simulink library "Word_Multiplexers_Lib"  (Simulink 8.7)
settings: Solver=ode45  StartTime=0.0  StopTime=10.0  RelTol=1e-3
(part 1 of 3)
settings Model: Creator=uzivatel  LastModifiedBy=Jozko Mrkvicka

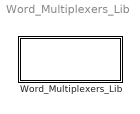
== system Word_Multiplexers_Lib ==
  Word_Multiplexers_Lib : Subsystem

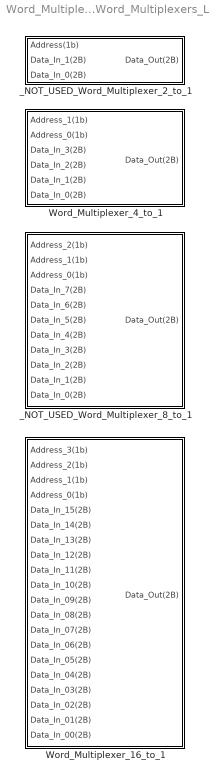
== system Word_Multiplexers_Lib/Word_Multiplexers_Lib ==
  Word_Multiplexer_16_to_1 : Subsystem
  Word_Multiplexer_4_to_1 : Subsystem
  _NOT_USED_Word_Multiplexer_2_to_1 : Subsystem
  _NOT_USED_Word_Multiplexer_8_to_1 : Subsystem
